simulink model "DrivetrainHevP2_SSC"  (R2022a)
settings: Solver=daessc  StartTime=0.0  StopTime=100  RelTol=1e-3
model workspace (MAT data in the model file):
  Aeff = 0.0314159265359
  Af = 2.27
  Apist_C0 = 0.0314159265359
  Apist_TCC = 0.001
  Bx = 10
  Cd = 0.25
  CoulFr_ShaftIn = 0
  Cx = 1.9
  DensAir = 1.293
  DerFac_C0 = 1
  DerFac_TCC = 1
  Drag_C0 = 0
  Drag_TCC = 0
  Dx = 1
  Eff_Diff = [0.98 0.98]
  Ex = 0.97
  FDrive = 3.32
  FZMAX = 6570
  FZMIN = 0
  G = [0 1 2 3 4 5 6]
  G_o = 1
  Iyy = 0.8
  Iyy_Whl = 0.8
  JCa_Diff = 0.001
  JEng = 0.01
  JMot = 0.21
  JPl_Diff = 0.001
  JShIn = 1e-05
  JShOut = 0.15
  Jd = 0.025
  Ji = 0.21
  Jin_Cltch = 0.2
  Jout = [0.009 0.01 0.01 0.01 0.01 0.01 0.01]
  Jout_Cltch = 0.01
  Jt = 0.01
  Jw1 = 0.01
  Jw2 = 0.01
  K_c = 10000
  KinFr_C0 = 0.4
  KinFr_TCC = 0.3
  Lrel = 0.15
  Mass = 1623
  N = [0.001 4.212 2.637 1.8 1.386 1 0.772]
  NF = 2
  NR = 2
  Ndiff = 3.32
  Ndisk = 1
  Neff_C0 = 1
  Neff_TCC = 6
  PEng_C0 = 30000
  PEng_TCC = 100
  Pabs = 101325
  Press = 300000
  PwrThr_Diff = [0.001 0.001]
  RatFr_ShaftIn = 1.1
  Re = 0.327
  Reff = 0.11
  Reff_C0 = 0.11
  Reff_TCC = 130
  Rm = 0.15
  SprStff_ShaftIn = 10000
  StatFr_C0 = 0.45
  StatFr_TCC = 0.35
  T = 273
  Temp_bpts = [313 358]
  Trq_bpts = [25 50 75 100 150 200 250]
  UNLOADED_RADIUS = 0.336
  VXLOW = 2
  VisFr_Diff = [0.001 0.001]
  ViscFr_ShaftIn = 400
  aMy = 0.01
  a_CG = 1.09
  alphaMy = 0
  b : Simulink.Parameter (value not decoded)
  bMy = 0
  b_CG = 1.7
  bd = 0.001
  betaMy = 1
  bi = 0.001
  bin_Cltch = 0.003
  bout = [0.003 0.003 0.003 0.003 0.003 0.003 0.003]
  bout_Cltch = 0.003
  br = 0.001
  bt = 0.001
  bw1 = 0.001
  bw2 = 0.001
  cMy = 0
  disk_abore = 0.05
  domega_o = 0
  eta = [0.95 0.95 0.95 0.95 0.95 0.95 0.95]
  eta_diff = 0.98
  eta_tbl = [1 1 1 1 1 1 1 1 1 1 1 1 ... (1078 elements, 7x11x7x2)]
  g = 9.81
  h = 0.5
  k : Simulink.Parameter (value not decoded)
  kappamax = 1.5
  lam_x = 1
  mu_kinetic = 0.35
  mu_static = 0.45
  muk = 0.4
  mus = 0.45
  num_pads = 2
  omega_bpts = [500.383141081 749.619781963 1002.67614148 1250.9578527 1499.23956393 1747.52127515 1995.80298637 2501.9157054 2998.47912785 4001.15526933 5003.83141081]
  omega_c : Simulink.Parameter (value not decoded)
  omega_o = 0
  omegai_o = 0
  omegal = 94.2477796077
  omegao = 0
  omegat_o = 0
  omegau = 83.7758040957
  omegaw1o = 0
  omegaw2o = 0
  phi = [0 0.5 0.6 0.7 0.8 0.87 0.92 0.94 0.96 0.97]
  phi_new = [0 0.5 0.6 0.7 0.8 0.87 0.92 0.94 0.96 0.97 0.99 1.02 ... (16 elements, 1x16)]
  philu = 0.85
  press = 700000
  psi = [12.2938 12.8588 13.1452 13.6285 14.6163 16.2675 19.3503 22.1046 29.9986 50]
  psi_new = [12.2938 12.8588 13.1452 13.6285 14.6163 16.2675 19.3503 22.1046 29.9986 50 48 41.76 ... (16 elements, 1x16)]
  tauC = 0.25
  tauTC = 0.1
  tau_s = 0.1
  theta_o = 0
  wc = 10
  win_o = 0
  wout_o = 0
  x_o = 0
  xdot_o = 0
  zeta = [2.232 1.5462 1.4058 1.2746 1.1528 1.0732 1.0192 0.9983 0.9983 0.9983]
  zeta_new = [2.232 1.5462 1.4058 1.2746 1.1528 1.0732 1.0192 0.9983 0.9983 0.9983 0.979797979798 1.04382929642 ... (16 elements, 1x16)]
libraries: fl_lib x66, nesl_utility x40, sdl_lib x25, simulink x7, autolibpowerinfoutils x5
(part 3 of 3)

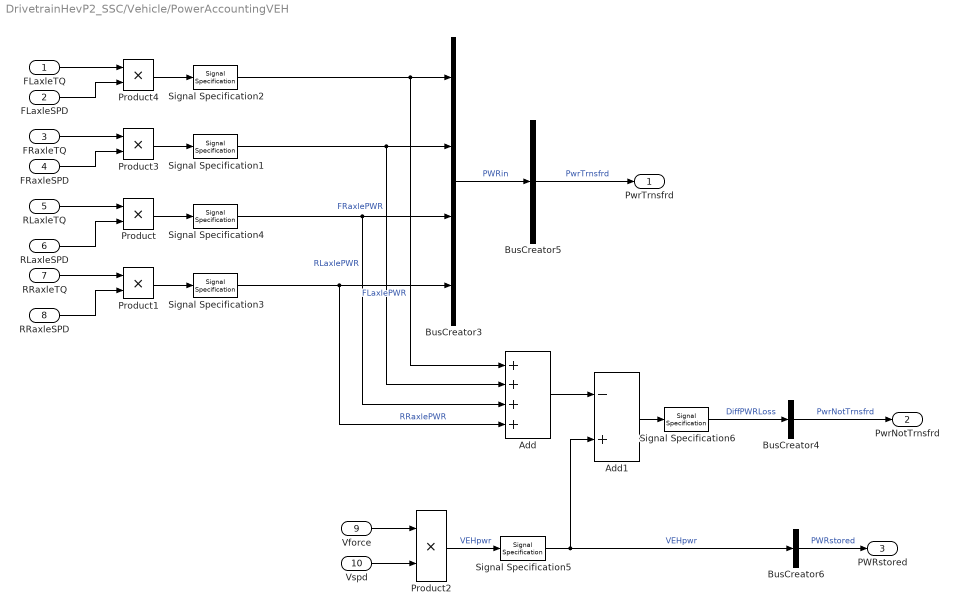
== system DrivetrainHevP2_SSC/Vehicle/PowerAccountingVEH ==
  FLaxleTQ : Inport
  FLaxleSPD : Inport  Port=2
  FRaxleTQ : Inport  Port=3
  FRaxleSPD : Inport  Port=4
  RLaxleTQ : Inport  Port=5
  RLaxleSPD : Inport  Port=6
  RRaxleTQ : Inport  Port=7
  RRaxleSPD : Inport  Port=8
  Vforce : Inport  Port=9
  Vspd : Inport  Port=10
  Add : Sum  Inputs=++++
  Add1 : Sum  Inputs=-+
  BusCreator3 : BusCreator  Inputs=4
  BusCreator4 : BusCreator  Inputs=1
  BusCreator5 : BusCreator  Inputs=1
  BusCreator6 : BusCreator  Inputs=1
  Product{,1..4} (5 alike) : Product
  Signal Specification{1..6} (6 alike) : SignalSpecification  Unit=W
  PwrTrnsfrd : Outport
  PwrNotTrnsfrd : Outport  Port=2
  PWRstored : Outport  Port=3
  wires:
  Signal Specification3/1 -> BusCreator3/4, Add/4  "RRaxlePWR"
  Signal Specification1/1 -> BusCreator3/2, Add/2  "FRaxlePWR"
  FRaxleTQ/1 -> Product3/1
  Signal Specification2/1 -> BusCreator3/1, Add/1  "FLaxlePWR"
  FRaxleSPD/1 -> Product3/2
  FLaxleTQ/1 -> Product4/1
  BusCreator3/1 -> BusCreator5/1  "PWRin"
  Product4/1 -> Signal Specification2/1
  Product3/1 -> Signal Specification1/1
  FLaxleSPD/1 -> Product4/2
  Product2/1 -> Signal Specification5/1  "VEHpwr"
  Product1/1 -> Signal Specification3/1
  Product/1 -> Signal Specification4/1
  Vspd/1 -> Product2/2
  Signal Specification4/1 -> BusCreator3/3, Add/3  "RLaxlePWR"
  RLaxleSPD/1 -> Product/2
  RRaxleTQ/1 -> Product1/1
  BusCreator5/1 -> PwrTrnsfrd/1  "PwrTrnsfrd"
  RRaxleSPD/1 -> Product1/2
  RLaxleTQ/1 -> Product/1
  BusCreator6/1 -> PWRstored/1  "PWRstored"
  Vforce/1 -> Product2/1
  Signal Specification6/1 -> BusCreator4/1  "DiffPWRLoss"
  BusCreator4/1 -> PwrNotTrnsfrd/1  "PwrNotTrnsfrd"
  Add1/1 -> Signal Specification6/1
  Add/1 -> Add1/1
  Signal Specification5/1 -> BusCreator6/1, Add1/2  "VEHpwr"

== system DrivetrainHevP2_SSC/Driveline/AWD/Subsystem ==
  Ideal Rotational Motion Sensor1 : fl_lib/Mechanical/Mechanical Sensors/Ideal Rotational Motion Sensor  wrap_angle=simscape.enum.onoff.off  offset=0 rad
      settings: SourceProductBaseCode=PW,SS,VE
  Ideal Torque Sensor2 : fl_lib/Mechanical/Mechanical Sensors/Ideal Torque Sensor
      settings: SourceProductBaseCode=PW,SS,VE
  Mechanical Rotational Reference1 : fl_lib/Mechanical/Rotational Elements/Mechanical Rotational Reference
      settings: SourceProductBaseCode=PW,SS,VE
  PS Terminator1 : fl_lib/Physical Signals/Sinks/PS Terminator
      settings: SourceProductBaseCode=PW,SS,VE
  PS-Simulink Converter3 : nesl_utility/PS-Simulink Converter  PhysicalDomain=network_engine_domain  SubClassName=ps_output  LeftPortType=input  RightPortType=output  PseudoPeriodic=off  Frequencies=[]  VectorFormat=1-D array  Unit=inherit  AffineConversion=off
      settings: SourceProductBaseCode=SS,PW,VE
  PS-Simulink Converter6 : nesl_utility/PS-Simulink Converter  PhysicalDomain=network_engine_domain  SubClassName=ps_output  LeftPortType=input  RightPortType=output  PseudoPeriodic=off  Frequencies=[]  VectorFormat=1-D array  Unit=inherit  AffineConversion=off
      settings: SourceProductBaseCode=SS,PW,VE
  Saturation1 : Saturate  UpperLimit=inf  LowerLimit=eps  ZeroCross=off
  C : PMIOPort  Side=Right
  R : PMIOPort  Port=2  Side=Left
  FRTrq : Outport
  FRSpd : Outport  Port=2
  wires:
  PS-Simulink Converter6/1 -> FRTrq/1  "FRTrq"
  Saturation1/1 -> FRSpd/1  "FRSpd"
  PS-Simulink Converter3/1 -> Saturation1/1
  connections:
  C/RConn1 -- Ideal Torque Sensor2/RConn1
  PS-Simulink Converter3/LConn1 -- Ideal Rotational Motion Sensor1/RConn2
  Mechanical Rotational Reference1/LConn1 -- Ideal Rotational Motion Sensor1/RConn1
  Ideal Rotational Motion Sensor1/LConn1 -- R/RConn1 -- Ideal Torque Sensor2/LConn1
  PS-Simulink Converter6/LConn1 -- Ideal Torque Sensor2/RConn2
  PS Terminator1/LConn1 -- Ideal Rotational Motion Sensor1/RConn3

== system DrivetrainHevP2_SSC/Driveline/AWD/Subsystem1 ==
  Ideal Rotational Motion Sensor1 : fl_lib/Mechanical/Mechanical Sensors/Ideal Rotational Motion Sensor  wrap_angle=simscape.enum.onoff.off  offset=0 rad
      settings: SourceProductBaseCode=PW,SS,VE
  Ideal Torque Sensor2 : fl_lib/Mechanical/Mechanical Sensors/Ideal Torque Sensor
      settings: SourceProductBaseCode=PW,SS,VE
  Mechanical Rotational Reference1 : fl_lib/Mechanical/Rotational Elements/Mechanical Rotational Reference
      settings: SourceProductBaseCode=PW,SS,VE
  PS Terminator1 : fl_lib/Physical Signals/Sinks/PS Terminator
      settings: SourceProductBaseCode=PW,SS,VE
  PS-Simulink Converter3 : nesl_utility/PS-Simulink Converter  PhysicalDomain=network_engine_domain  SubClassName=ps_output  LeftPortType=input  RightPortType=output  PseudoPeriodic=off  Frequencies=[]  VectorFormat=1-D array  Unit=inherit  AffineConversion=off
      settings: SourceProductBaseCode=SS,PW,VE
  PS-Simulink Converter6 : nesl_utility/PS-Simulink Converter  PhysicalDomain=network_engine_domain  SubClassName=ps_output  LeftPortType=input  RightPortType=output  PseudoPeriodic=off  Frequencies=[]  VectorFormat=1-D array  Unit=inherit  AffineConversion=off
      settings: SourceProductBaseCode=SS,PW,VE
  Saturation1 : Saturate  UpperLimit=inf  LowerLimit=eps  ZeroCross=off
  C : PMIOPort  Side=Right
  R : PMIOPort  Port=2  Side=Left
  FLTrq : Outport
  FLSpd : Outport  Port=2
  wires:
  PS-Simulink Converter6/1 -> FLTrq/1  "FLTrq"
  Saturation1/1 -> FLSpd/1  "FLSpd"
  PS-Simulink Converter3/1 -> Saturation1/1
  connections:
  C/RConn1 -- Ideal Torque Sensor2/RConn1
  PS-Simulink Converter3/LConn1 -- Ideal Rotational Motion Sensor1/RConn2
  Mechanical Rotational Reference1/LConn1 -- Ideal Rotational Motion Sensor1/RConn1
  R/RConn1 -- Ideal Torque Sensor2/LConn1 -- Ideal Rotational Motion Sensor1/LConn1
  PS-Simulink Converter6/LConn1 -- Ideal Torque Sensor2/RConn2
  PS Terminator1/LConn1 -- Ideal Rotational Motion Sensor1/RConn3

== system DrivetrainHevP2_SSC/Driveline/AWD/Subsystem2 ==
  Ideal Rotational Motion Sensor1 : fl_lib/Mechanical/Mechanical Sensors/Ideal Rotational Motion Sensor  wrap_angle=simscape.enum.onoff.off  offset=0 rad
      settings: SourceProductBaseCode=PW,SS,VE
  Ideal Torque Sensor2 : fl_lib/Mechanical/Mechanical Sensors/Ideal Torque Sensor
      settings: SourceProductBaseCode=PW,SS,VE
  Mechanical Rotational Reference1 : fl_lib/Mechanical/Rotational Elements/Mechanical Rotational Reference
      settings: SourceProductBaseCode=PW,SS,VE
  PS Terminator1 : fl_lib/Physical Signals/Sinks/PS Terminator
      settings: SourceProductBaseCode=PW,SS,VE
  PS-Simulink Converter3 : nesl_utility/PS-Simulink Converter  PhysicalDomain=network_engine_domain  SubClassName=ps_output  LeftPortType=input  RightPortType=output  PseudoPeriodic=off  Frequencies=[]  VectorFormat=1-D array  Unit=inherit  AffineConversion=off
      settings: SourceProductBaseCode=SS,PW,VE
  PS-Simulink Converter6 : nesl_utility/PS-Simulink Converter  PhysicalDomain=network_engine_domain  SubClassName=ps_output  LeftPortType=input  RightPortType=output  PseudoPeriodic=off  Frequencies=[]  VectorFormat=1-D array  Unit=inherit  AffineConversion=off
      settings: SourceProductBaseCode=SS,PW,VE
  Saturation1 : Saturate  UpperLimit=inf  LowerLimit=eps  ZeroCross=off
  C : PMIOPort  Side=Right
  R : PMIOPort  Port=2  Side=Left
  RLTrq : Outport
  RLSpd : Outport  Port=2
  wires:
  PS-Simulink Converter6/1 -> RLTrq/1  "FRTrq"
  Saturation1/1 -> RLSpd/1  "FRSpd"
  PS-Simulink Converter3/1 -> Saturation1/1
  connections:
  C/RConn1 -- Ideal Torque Sensor2/RConn1
  PS-Simulink Converter3/LConn1 -- Ideal Rotational Motion Sensor1/RConn2
  Mechanical Rotational Reference1/LConn1 -- Ideal Rotational Motion Sensor1/RConn1
  R/RConn1 -- Ideal Torque Sensor2/LConn1 -- Ideal Rotational Motion Sensor1/LConn1
  PS-Simulink Converter6/LConn1 -- Ideal Torque Sensor2/RConn2
  PS Terminator1/LConn1 -- Ideal Rotational Motion Sensor1/RConn3

== system DrivetrainHevP2_SSC/Driveline/AWD/Subsystem3 ==
  Ideal Rotational Motion Sensor1 : fl_lib/Mechanical/Mechanical Sensors/Ideal Rotational Motion Sensor  wrap_angle=simscape.enum.onoff.off  offset=0 rad
      settings: SourceProductBaseCode=PW,SS,VE
  Ideal Torque Sensor2 : fl_lib/Mechanical/Mechanical Sensors/Ideal Torque Sensor
      settings: SourceProductBaseCode=PW,SS,VE
  Mechanical Rotational Reference1 : fl_lib/Mechanical/Rotational Elements/Mechanical Rotational Reference
      settings: SourceProductBaseCode=PW,SS,VE
  PS Terminator1 : fl_lib/Physical Signals/Sinks/PS Terminator
      settings: SourceProductBaseCode=PW,SS,VE
  PS-Simulink Converter3 : nesl_utility/PS-Simulink Converter  PhysicalDomain=network_engine_domain  SubClassName=ps_output  LeftPortType=input  RightPortType=output  PseudoPeriodic=off  Frequencies=[]  VectorFormat=1-D array  Unit=inherit  AffineConversion=off
      settings: SourceProductBaseCode=SS,PW,VE
  PS-Simulink Converter6 : nesl_utility/PS-Simulink Converter  PhysicalDomain=network_engine_domain  SubClassName=ps_output  LeftPortType=input  RightPortType=output  PseudoPeriodic=off  Frequencies=[]  VectorFormat=1-D array  Unit=inherit  AffineConversion=off
      settings: SourceProductBaseCode=SS,PW,VE
  Saturation1 : Saturate  UpperLimit=inf  LowerLimit=eps  ZeroCross=off
  C : PMIOPort  Side=Right
  R : PMIOPort  Port=2  Side=Left
  RRTrq : Outport
  RRSpd : Outport  Port=2
  wires:
  PS-Simulink Converter3/1 -> Saturation1/1
  Saturation1/1 -> RRSpd/1  "FRSpd"
  PS-Simulink Converter6/1 -> RRTrq/1  "FRTrq"
  connections:
  PS Terminator1/LConn1 -- Ideal Rotational Motion Sensor1/RConn3
  PS-Simulink Converter6/LConn1 -- Ideal Torque Sensor2/RConn2
  Ideal Rotational Motion Sensor1/LConn1 -- Ideal Torque Sensor2/LConn1 -- R/RConn1
  Mechanical Rotational Reference1/LConn1 -- Ideal Rotational Motion Sensor1/RConn1
  PS-Simulink Converter3/LConn1 -- Ideal Rotational Motion Sensor1/RConn2
  C/RConn1 -- Ideal Torque Sensor2/RConn1

== system DrivetrainHevP2_SSC/Driveline/FWD/Subsystem ==
  Ideal Rotational Motion Sensor1 : fl_lib/Mechanical/Mechanical Sensors/Ideal Rotational Motion Sensor  wrap_angle=simscape.enum.onoff.off  offset=0 rad
      settings: SourceProductBaseCode=PW,SS,VE
  Ideal Torque Sensor2 : fl_lib/Mechanical/Mechanical Sensors/Ideal Torque Sensor
      settings: SourceProductBaseCode=PW,SS,VE
  Mechanical Rotational Reference1 : fl_lib/Mechanical/Rotational Elements/Mechanical Rotational Reference
      settings: SourceProductBaseCode=PW,SS,VE
  PS Terminator1 : fl_lib/Physical Signals/Sinks/PS Terminator
      settings: SourceProductBaseCode=PW,SS,VE
  PS-Simulink Converter3 : nesl_utility/PS-Simulink Converter  PhysicalDomain=network_engine_domain  SubClassName=ps_output  LeftPortType=input  RightPortType=output  PseudoPeriodic=off  Frequencies=[]  VectorFormat=1-D array  Unit=inherit  AffineConversion=off
      settings: SourceProductBaseCode=SS,PW,VE
  PS-Simulink Converter6 : nesl_utility/PS-Simulink Converter  PhysicalDomain=network_engine_domain  SubClassName=ps_output  LeftPortType=input  RightPortType=output  PseudoPeriodic=off  Frequencies=[]  VectorFormat=1-D array  Unit=inherit  AffineConversion=off
      settings: SourceProductBaseCode=SS,PW,VE
  Saturation1 : Saturate  UpperLimit=inf  LowerLimit=eps  ZeroCross=off
  C : PMIOPort  Side=Right
  R : PMIOPort  Port=2  Side=Left
  FRTrq : Outport
  FRSpd : Outport  Port=2
  wires:
  PS-Simulink Converter3/1 -> Saturation1/1
  Saturation1/1 -> FRSpd/1  "FRSpd"
  PS-Simulink Converter6/1 -> FRTrq/1  "FRTrq"
  connections:
  PS Terminator1/LConn1 -- Ideal Rotational Motion Sensor1/RConn3
  PS-Simulink Converter6/LConn1 -- Ideal Torque Sensor2/RConn2
  Ideal Torque Sensor2/LConn1 -- R/RConn1 -- Ideal Rotational Motion Sensor1/LConn1
  Mechanical Rotational Reference1/LConn1 -- Ideal Rotational Motion Sensor1/RConn1
  PS-Simulink Converter3/LConn1 -- Ideal Rotational Motion Sensor1/RConn2
  C/RConn1 -- Ideal Torque Sensor2/RConn1

== system DrivetrainHevP2_SSC/Driveline/FWD/Subsystem1 ==
  Ideal Rotational Motion Sensor1 : fl_lib/Mechanical/Mechanical Sensors/Ideal Rotational Motion Sensor  wrap_angle=simscape.enum.onoff.off  offset=0 rad
      settings: SourceProductBaseCode=PW,SS,VE
  Ideal Torque Sensor2 : fl_lib/Mechanical/Mechanical Sensors/Ideal Torque Sensor
      settings: SourceProductBaseCode=PW,SS,VE
  Mechanical Rotational Reference1 : fl_lib/Mechanical/Rotational Elements/Mechanical Rotational Reference
      settings: SourceProductBaseCode=PW,SS,VE
  PS Terminator1 : fl_lib/Physical Signals/Sinks/PS Terminator
      settings: SourceProductBaseCode=PW,SS,VE
  PS-Simulink Converter3 : nesl_utility/PS-Simulink Converter  PhysicalDomain=network_engine_domain  SubClassName=ps_output  LeftPortType=input  RightPortType=output  PseudoPeriodic=off  Frequencies=[]  VectorFormat=1-D array  Unit=inherit  AffineConversion=off
      settings: SourceProductBaseCode=SS,PW,VE
  PS-Simulink Converter6 : nesl_utility/PS-Simulink Converter  PhysicalDomain=network_engine_domain  SubClassName=ps_output  LeftPortType=input  RightPortType=output  PseudoPeriodic=off  Frequencies=[]  VectorFormat=1-D array  Unit=inherit  AffineConversion=off
      settings: SourceProductBaseCode=SS,PW,VE
  Saturation1 : Saturate  UpperLimit=inf  LowerLimit=eps  ZeroCross=off
  C : PMIOPort  Side=Right
  R : PMIOPort  Port=2  Side=Left
  FRTrq : Outport
  FRSpd : Outport  Port=2
  wires:
  PS-Simulink Converter3/1 -> Saturation1/1
  Saturation1/1 -> FRSpd/1  "FRSpd"
  PS-Simulink Converter6/1 -> FRTrq/1  "FRTrq"
  connections:
  PS Terminator1/LConn1 -- Ideal Rotational Motion Sensor1/RConn3
  PS-Simulink Converter6/LConn1 -- Ideal Torque Sensor2/RConn2
  Ideal Rotational Motion Sensor1/LConn1 -- Ideal Torque Sensor2/LConn1 -- R/RConn1
  Mechanical Rotational Reference1/LConn1 -- Ideal Rotational Motion Sensor1/RConn1
  PS-Simulink Converter3/LConn1 -- Ideal Rotational Motion Sensor1/RConn2
  C/RConn1 -- Ideal Torque Sensor2/RConn1

== system DrivetrainHevP2_SSC/Transmission/Actuator/Actuator dynamics ==
  In : Inport
  Gain : Gain  Gain=1./b
  Integrator : Integrator  InitialCondition=[0 0 0 0 0].*b
  Sum : Sum  Inputs=|+-  InputSameDT=on  SaturateOnIntegerOverflow=on  OutDataTypeStr=Inherit: Same as first input
  Out : Outport  VectorParamsAs1DForOutWhenUnconnected=off
  wires:
  Sum/1 -> Integrator/1
  In/1 -> Sum/1
  Integrator/1 -> Gain/1
  Gain/1 -> Sum/2, Out/1
